simulink model "bmi_auto_calibration_tester"  (R2023b)
settings: Solver=VariableStepAuto  StartTime=0.0  StopTime=671  RelTol=1e-3
libraries: dspstat3 x1, matrix_library x1, vrlib x1
settings Model: Creator=TAK  LastModifiedBy=Inver
settings DataIOCC: ExternalInput=Sheet1.getElement('accel_x'),Sheet1.getElement('accel_y'),Sheet1.getElement('accel_z'),Sheet1.getElement('gyro_x'),Sheet1.getElement('gyro_y'),Sheet1.getElement('gyro_z'),Sheet1.getElement('hv_on'),Sheet1.getElement('rtd')  LoadExternalInput=on

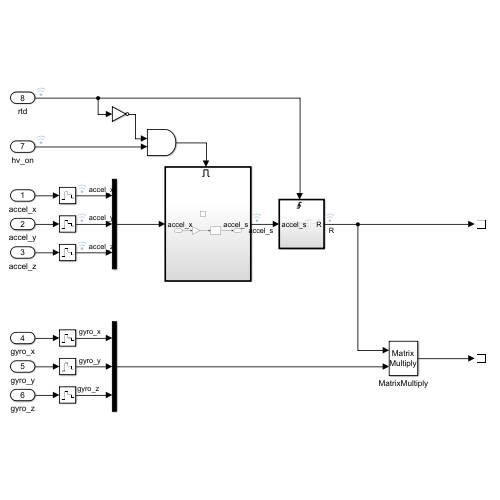
[thumbnail: Simulink's stored preview of the top-level diagram]
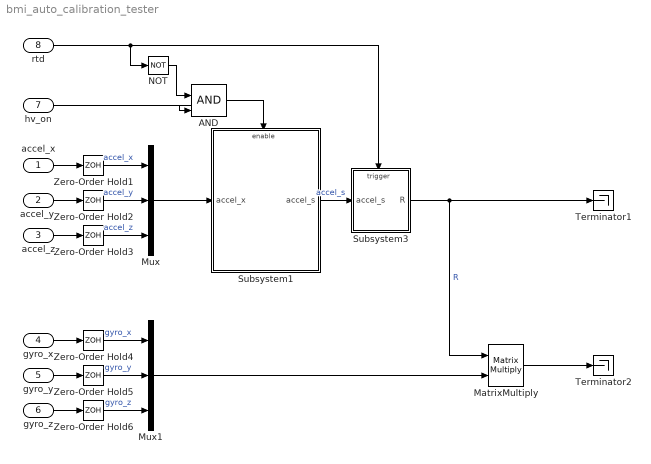
== system bmi_auto_calibration_tester ==
  accel_x : Inport  PortDimensions=1
  accel_y : Inport  Port=2  PortDimensions=1
  accel_z : Inport  Port=3  PortDimensions=1
  gyro_x : Inport  Port=4  PortDimensions=1
  gyro_y : Inport  Port=5  PortDimensions=1
  gyro_z : Inport  Port=6  PortDimensions=1
  hv_on : Inport  Port=7
  rtd : Inport  Port=8
  AND : Logic  IconShape=distinctive  AllPortsSameDT=off  OutDataTypeStr=boolean
  MatrixMultiply : Product  Multiplication=Matrix(*)
  Mux : Mux  Inputs=3
  Mux1 : Mux  Inputs=3
  NOT : Logic  Operator=NOT  IconShape=distinctive  AllPortsSameDT=off  OutDataTypeStr=boolean
  Subsystem1 : Subsystem
  Subsystem3 : Subsystem
  Terminator1 : Terminator
  Terminator2 : Terminator
  Zero-Order Hold{1..6} (6 alike) : ZeroOrderHold  SampleTime=.02
  wires:
  accel_x/1 -> Zero-Order Hold1/1
  accel_y/1 -> Zero-Order Hold2/1
  accel_z/1 -> Zero-Order Hold3/1
  gyro_x/1 -> Zero-Order Hold4/1
  gyro_y/1 -> Zero-Order Hold5/1
  gyro_z/1 -> Zero-Order Hold6/1
  Subsystem1/1(accel_s) -> Subsystem3/1(accel_s)  "accel_s"
  Subsystem3/1(R) -> MatrixMultiply/1, Terminator1/1  "R"
  AND/1 -> Subsystem1/Enable
  rtd/1 -> NOT/1, Subsystem3/Trigger
  NOT/1 -> AND/1
  hv_on/1 -> AND/2
  Zero-Order Hold1/1 -> Mux/1  "accel_x"
  Zero-Order Hold2/1 -> Mux/2  "accel_y"
  Zero-Order Hold3/1 -> Mux/3  "accel_z"
  Zero-Order Hold4/1 -> Mux1/1  "gyro_x"
  Zero-Order Hold5/1 -> Mux1/2  "gyro_y"
  Zero-Order Hold6/1 -> Mux1/3  "gyro_z"
  Mux/1 -> Subsystem1/1(accel_x)
  Mux1/1 -> MatrixMultiply/2
  MatrixMultiply/1 -> Terminator2/1

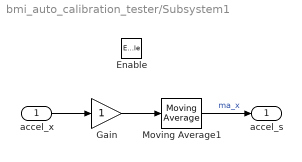
== system bmi_auto_calibration_tester/Subsystem1 ==
  accel_x : Inport
  Enable : EnablePort
  Gain : Gain
  Moving Average1 : dspstat3/Moving Average  Method=Sliding window  ForgettingFactorPort=off  SpecifyWindowLength=off  WindowLength=4  OverlapLength=3  AllowArbitraryInputLength=off  ForgettingFactor=0.9  SimulateUsing=Code generation
  accel_s : Outport
  wires:
  Moving Average1/1 -> accel_s/1  "ma_x"
  Gain/1 -> Moving Average1/1
  accel_x/1 -> Gain/1

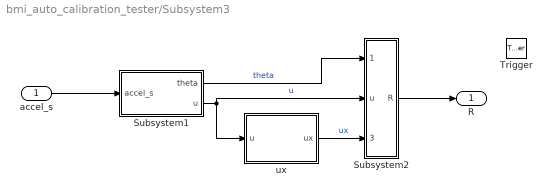
== system bmi_auto_calibration_tester/Subsystem3 ==
  accel_s : Inport
  Trigger : TriggerPort  VariantControl=(inherit)  PortDimensions=1
  Subsystem1 : Subsystem
  Subsystem2 : Subsystem
  ux : MATLAB Function  TreatAsAtomicUnit=on
  R : Outport
  wires:
  ux/1(ux) -> Subsystem2/3(ux)  "ux"
  Subsystem1/2(u) -> ux/1(u), Subsystem2/2(u)  "u"
  Subsystem1/1(theta) -> Subsystem2/1(theta)  "theta"
  Subsystem2/1(R) -> R/1
  accel_s/1 -> Subsystem1/1(accel_s)

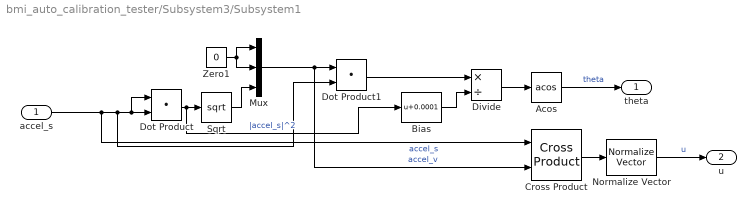
== system bmi_auto_calibration_tester/Subsystem3/Subsystem1 ==
  accel_s : Inport  PortDimensions=[3 1]
  Acos : Trigonometry  Operator=acos
  Bias : Bias  Bias=0.0001  SaturateOnIntegerOverflow=off
  Cross Product : matrix_library/Cross Product
  Divide : Product  Inputs=*/
  Dot Product : DotProduct  OutDataTypeStr=Inherit: Inherit via internal rule
  Dot Product1 : DotProduct  OutDataTypeStr=Inherit: Inherit via internal rule
  Mux : Mux  Inputs=3
  Normalize Vector : vrlib/Utilities/Normalize Vector  maxzero=0
  Sqrt : Sqrt
  Zero1 : Constant  Value=0  OutDataTypeStr=Inherit: Inherit via back propagation
  theta : Outport
  u : Outport  Port=2
  wires:
  accel_s/1 -> Cross Product/1, Dot Product1/2, Dot Product/1, Dot Product/2  "accel_s"
  Cross Product/1 -> Normalize Vector/1
  Dot Product1/1 -> Divide/1
  Normalize Vector/1 -> u/1  "u"
  Dot Product/1 -> Bias/1, Sqrt/1  "|accel_s|^2"
  Sqrt/1 -> Mux/3
  Mux/1 -> Cross Product/2, Dot Product1/1  "accel_v"
  Zero1/1 -> Mux/1, Mux/2
  Divide/1 -> Acos/1
  Acos/1 -> theta/1  "theta"
  Bias/1 -> Divide/2

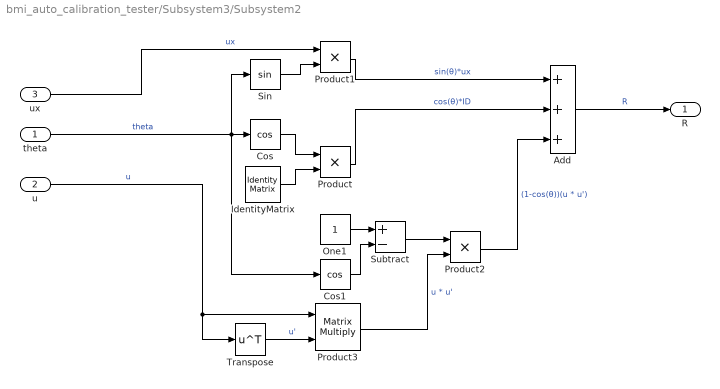
== system bmi_auto_calibration_tester/Subsystem3/Subsystem2 ==
  theta : Inport
  u : Inport  Port=2
  ux : Inport  Port=3
  Add : Sum  Inputs=+++
  Cos : Trigonometry  Operator=cos
  Cos1 : Trigonometry  Operator=cos
  IdentityMatrix : IdentityMatrix  OutputDimensions=3  SampleTime=-1
  One1 : Constant  OutDataTypeStr=Inherit: Inherit via back propagation
  Product : Product
  Product1 : Product
  Product2 : Product
  Product3 : Product  Multiplication=Matrix(*)
  Sin : Trigonometry
  Subtract : Sum  Inputs=+-
  Transpose : Math  Operator=transpose
  R : Outport
  wires:
  theta/1 -> Cos1/1, Sin/1, Cos/1  "theta"
  Product/1 -> Add/2  "cos(θ)*ID"
  Cos1/1 -> Subtract/2
  Cos/1 -> Product/1
  Subtract/1 -> Product2/1
  ux/1 -> Product1/1  "ux"
  One1/1 -> Subtract/1
  IdentityMatrix/1 -> Product/2
  u/1 -> Product3/1, Transpose/1  "u"
  Sin/1 -> Product1/2
  Product1/1 -> Add/1  "sin(θ)*ux"
  Add/1 -> R/1  "R"
  Transpose/1 -> Product3/2  "u'"
  Product2/1 -> Add/3  "(1-cos(θ))(u * u')"
  Product3/1 -> Product2/2  "u * u'"

== matlab function bmi_auto_calibration_tester/Subsystem3/ux ==
  data: u input size=[3 1]; ux output
function ux = fcn(u)

ux = [0 -u(3) u(2); u(3) 0 -u(1); -u(2) u(1) 0];
